simulink model "IP_FOC"  (R2020a)
settings: Solver=ode113  StartTime=0.0  StopTime=10  FixedStep=1e-4  RelTol=1e-4
settings Model: Creator=LENOVO PC  LastModifiedBy=LENOVO PC
settings DataIOCC: ReturnWorkspaceOutputs=off

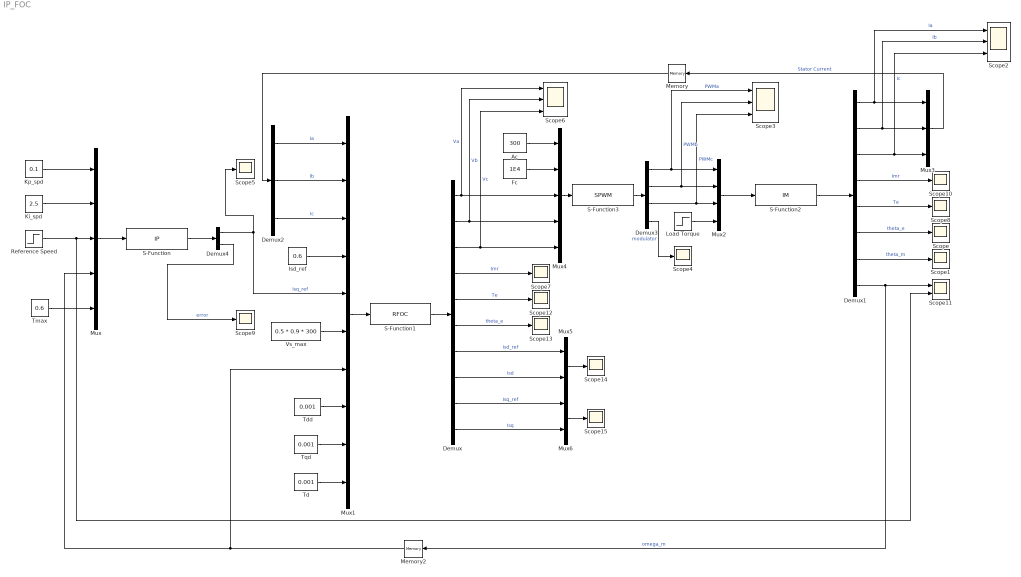
== system IP_FOC ==
  Ac : Constant  Value=300
  Demux : Demux  Outputs=10
  Demux1 : Demux  Outputs=8
  Demux2 : Demux  Outputs=3
  Demux3 : Demux
  Demux4 : Demux  Outputs=2
  Fc : Constant  Value=1E4
  Isd_ref : Constant  Value=0.6
  Ki_spd : Constant  Value=2.5
  Kp_spd : Constant  Value=0.1
  Load Torque : Step  Time=0  After=0  SampleTime=0
  Memory : Memory
  Memory2 : Memory
  Mux : Mux  Inputs=5
  Mux1 : Mux  Inputs=10
  Mux2 : Mux
  Mux3 : Mux  Inputs=3
  Mux4 : Mux  Inputs=5
  Mux5 : Mux  Inputs=2
  Mux6 : Mux  Inputs=2
  Reference Speed : Step  Time=0  After=100  SampleTime=0
  S-Function : S-Function  FunctionName=IP  SFunctionDeploymentMode=off  EnableBusSupport=off
  S-Function1 : S-Function  FunctionName=RFOC  SFunctionDeploymentMode=off  EnableBusSupport=off
  S-Function2 : S-Function  FunctionName=IM  SFunctionDeploymentMode=off  EnableBusSupport=off
  S-Function3 : S-Function  FunctionName=SPWM  SFunctionDeploymentMode=off  EnableBusSupport=off
  Scope{,1,4..5,7..10,12..15} (12 alike) : Scope
  Scope11 : Scope  NumInputPorts=2
  Scope2 : Scope  NumInputPorts=3
  Scope3 : Scope  NumInputPorts=3
  Scope6 : Scope  NumInputPorts=3
  Td : Constant  Value=0.001
  Tdd : Constant  Value=0.001
  Tmax : Constant  Value=0.6
  Tqd : Constant  Value=0.001
  Vs_max : Constant  Value=0.5 * 0.9 * 300
  wires:
  Mux/1 -> S-Function/1
  Ki_spd/1 -> Mux/2
  Memory2/1 -> Mux1/7, Mux/4
  Memory/1 -> Demux2/1
  Mux2/1 -> S-Function2/1
  Demux1/3 -> Scope2/3, Mux3/3  "Ic"
  Ac/1 -> Mux4/1
  Demux2/1 -> Mux1/1  "Ia"
  Demux2/2 -> Mux1/2  "Ib"
  Mux3/1 -> Memory/1  "Stator Current"
  Demux1/2 -> Scope2/2, Mux3/2  "Ib"
  S-Function2/1 -> Demux1/1
  Kp_spd/1 -> Mux/1
  Demux1/1 -> Mux3/1, Scope2/1  "Ia"
  Load Torque/1 -> Mux2/4
  Demux2/3 -> Mux1/3  "Ic"
  S-Function1/1 -> Demux/1
  Mux1/1 -> S-Function1/1
  Demux1/6 -> Scope/1  "theta_e"
  Demux1/7 -> Scope1/1  "theta_m"
  Demux1/5 -> Scope8/1  "Te"
  Demux1/8 -> Memory2/1, Scope11/1  "omega_m"
  Fc/1 -> Mux4/2
  Demux3/1 -> Mux2/1, Scope3/1  "PWMa"
  Demux3/2 -> Mux2/2, Scope3/2  "PWMb"
  Demux3/3 -> Scope3/3, Mux2/3  "PWMc"
  Demux3/4 -> Scope4/1  "modulator"
  Demux/1 -> Scope6/1, Mux4/3  "Va"
  Demux/2 -> Scope6/2, Mux4/4  "Vb"
  Demux/3 -> Scope6/3, Mux4/5  "Vc"
  S-Function/1 -> Demux4/1
  Demux4/1 -> Scope5/1, Mux1/5  "Isq_ref"
  Demux4/2 -> Scope9/1  "error"
  Reference Speed/1 -> Mux/3, Scope11/2
  Demux1/4 -> Scope10/1  "Imr"
  Demux/4 -> Scope7/1  "Imr"
  Demux/5 -> Scope12/1  "Te"
  Demux/6 -> Scope13/1  "theta_e"
  Demux/7 -> Mux5/1  "Isd_ref"
  Demux/8 -> Mux5/2  "Isd"
  Demux/9 -> Mux6/1  "Isq_ref"
  Demux/10 -> Mux6/2  "Isq"
  Mux5/1 -> Scope14/1
  Mux6/1 -> Scope15/1
  Vs_max/1 -> Mux1/6
  Mux4/1 -> S-Function3/1
  S-Function3/1 -> Demux3/1
  Tdd/1 -> Mux1/8
  Tqd/1 -> Mux1/9
  Td/1 -> Mux1/10
  Isd_ref/1 -> Mux1/4
  Tmax/1 -> Mux/5
